simulink model "positionCtrlEmulatorTest"  (Simulink 9.0)
settings: Solver=FixedStepDiscrete  StartTime=0.0  StopTime=CONFIG.Tend  FixedStep=CONFIG.Ts  RelTol=1e-3
InitFcn:
  | positionCtrlEmulatorTestInit
undefined symbols (not defined in the file or in its folder): CONFIG, DiscIntNeverNeededParam
libraries: WBToolboxLibrary x6
settings Model: SuppressorTable=22 serialization::archive 11 0 6 0 0 0 0 0  Creator=nunoguedelha  LastModifiedBy=nunoguedelha
settings DataIOCC: SaveFormat=Dataset
settings OptimizationCC: LifeSpan=auto
settings DebuggingCC: UnderspecifiedInitializationDetection=Simplified  MergeDetectMultiDrivingBlocksExec=error  SFUnexpectedBacktrackingDiag=error  SFNoUnconditionalDefaultTransitionDiag=error  SFExecutionAtInitializationDiag=warning
settings HardwareCC: ProdBitPerPointer=64  ProdBitPerSizeT=64  ProdBitPerPtrDiffT=64  ProdLargestAtomicFloat=Float  ProdIntDivRoundTo=Zero  ProdEndianess=LittleEndian  ProdWordSize=64  ProdHWDeviceType=Intel->x86-64 (Windows64)
settings ModelReferenceCC: PropagateSignalLabelsOutOfModel=on
settings CodeAppCC: StateflowObjectComments=off
settings GRTTargetCC: TargetLangStandard=C99 (ISO)
settings ConfigComp: CovMetricSettings=dwe  CovHtmlReporting=off  CovSaveCumulativeToWorkspaceVar=off  CovSaveSingleToWorkspaceVar=off  CovExternalEMLEnable=on

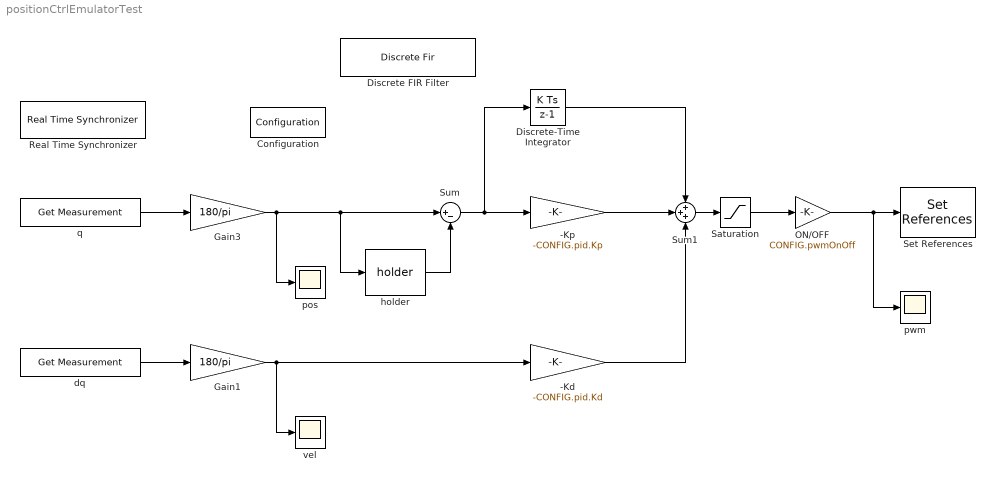
== system positionCtrlEmulatorTest ==
  -Kd : Gain  Gain=-CONFIG.pid.Kd
  -Kp : Gain  Gain=-CONFIG.pid.Kp
  Configuration : WBToolboxLibrary/Utilities/Configuration  ConfigSource=Mask  ConfigObject='WBTConfigRobot'  RobotName='icub'  UrdfFile='model.urdf'  ControlledJoints=CONFIG.ctrledJoints  ControlBoardsNames=CONFIG.ctrlBoards  LocalName='WBT'  GravityVector=[0,0,-9.81]
      settings: SourceProductName=Whole Body Toolbox
  Discrete FIR Filter : DiscreteFir  Coefficients=[0.4 0.3 0.2 0.1]  SampleTime=CONFIG.Ts
  Discrete-Time Integrator : DiscreteIntegrator  gainval=-CONFIG.pid.Ki  InitialCondition=zeros(CONFIG.jointsDoF,1)  InitialConditionSetting=State (most efficient)  SampleTime=CONFIG.Ts  LimitOutput=on  UpperSaturationLimit=CONFIG.pid.IntLimit  LowerSaturationLimit=-CONFIG.pid.IntLimit  ICPrevOutput=DiscIntNeverNeededParam  ICPrevScaledInput=DiscIntNeverNeededParam
  Gain1 : Gain  Gain=180/pi
  Gain3 : Gain  Gain=180/pi
  ON/OFF : Gain  Gain=CONFIG.pwmOnOff
  Real Time Synchronizer : WBToolboxLibrary/Utilities/Real Time Synchronizer  period=CONFIG.Ts
      settings: SourceProductName=Whole Body Toolbox
  Saturation : Saturate  UpperLimit=CONFIG.pid.outLimit  LowerLimit=-CONFIG.pid.outLimit
  Set References : WBToolboxLibrary/wholeBodyActuators/Set References  controlType=PWM  refSpeed=50
      settings: SourceProductName=Whole Body Toolbox
  Sum : Sum  Inputs=|+-
  Sum1 : Sum  Inputs=+++
  dq : WBToolboxLibrary/wholeBodyStates/Get Measurement  measuredType=Joints Velocity
      settings: SourceProductName=Whole Body Toolbox
  "holder " : WBToolboxLibrary/Utilities/holder 
      settings: SourceProductName=Whole Body Toolbox
  pos : Scope
  pwm : Scope
  q : WBToolboxLibrary/wholeBodyStates/Get Measurement  measuredType=Joints Position
      settings: SourceProductName=Whole Body Toolbox
  vel : Scope
  wires:
  q/1 -> Gain3/1
  "holder "/1 -> Sum/2
  Gain3/1 -> pos/1, "holder "/1, Sum/1
  Sum1/1 -> Saturation/1
  Saturation/1 -> ON/OFF/1
  ON/OFF/1 -> pwm/1, Set References/1
  -Kd/1 -> Sum1/3
  -Kp/1 -> Sum1/2
  Sum/1 -> Discrete-Time Integrator/1, -Kp/1
  Gain1/1 -> -Kd/1, vel/1
  dq/1 -> Gain1/1
  Discrete-Time Integrator/1 -> Sum1/1
